simulink model "Outer_Loop_Autopilot"  (R2021b)
settings: Solver=FixedStepAuto  StartTime=0.0  StopTime=10.0  FixedStep=0.01  RelTol=1e-3
undefined symbols (not defined in the file): ap, uavParam
libraries: simulink x3, slpidlib x2, simulink_need_slupdate x1
settings Model: DataDictionary=stepFideltyResponseData.sldd  ModifiedByFormat=The MathWorks, Inc.  Creator=The MathWorks, Inc.  LastModifiedBy=The MathWorks, Inc.
settings DataIOCC: SaveOutput=off  SaveTime=off
settings OptimizationCC: UseDivisionForNetSlopeComputation=UseDivisionForReciprocalsOfIntegersOnly

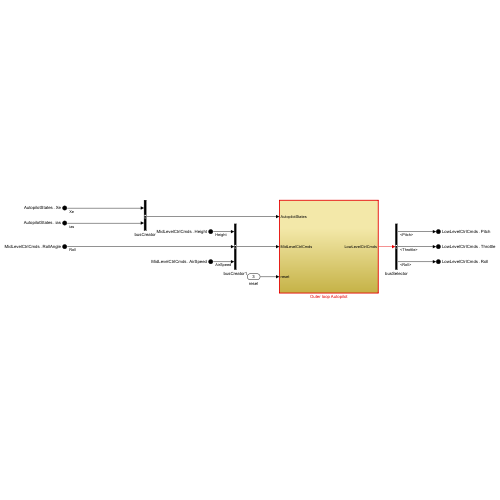
[thumbnail: Simulink's stored preview of the top-level diagram]
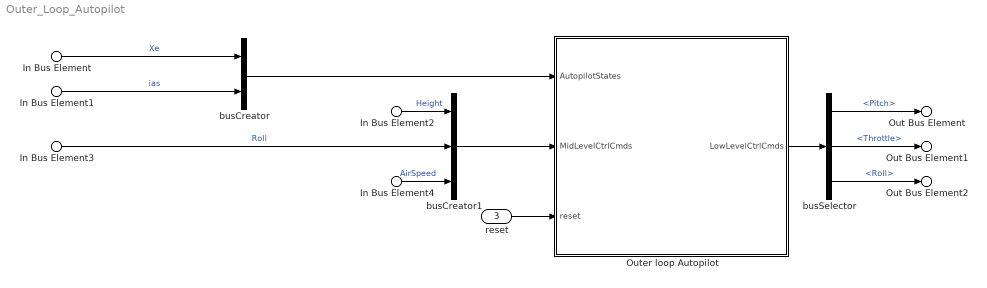
== system Outer_Loop_Autopilot ==
  In Bus Element : Inport  PortName=AutopilotStates  Element=Xe
  In Bus Element1 : Inport  PortName=AutopilotStates  Element=ias
  In Bus Element2 : Inport  Port=2  PortName=MidLevelCtrlCmds  Element=Height
  In Bus Element3 : Inport  Port=2  PortName=MidLevelCtrlCmds  Element=RollAngle
  In Bus Element4 : Inport  Port=2  PortName=MidLevelCtrlCmds  Element=AirSpeed
  reset : Inport  Port=3  OutDataTypeStr=double  PortDimensions=1  SampleTime=[0.01,0]
  Outer loop Autopilot : Subsystem  TreatAsAtomicUnit=on
  busCreator : BusCreator  Inputs=2
  busCreator1 : BusCreator  Inputs=3
  busSelector : BusSelector  OutputSignals=Pitch,Throttle,Roll
  Out Bus Element : Outport  PortName=LowLevelCtrlCmds  Element=Pitch
  Out Bus Element1 : Outport  PortName=LowLevelCtrlCmds  Element=Throttle
  Out Bus Element2 : Outport  PortName=LowLevelCtrlCmds  Element=Roll
  wires:
  busCreator1/1 -> Outer loop Autopilot/2(MidLevelCtrlCmds)
  Outer loop Autopilot/1(LowLevelCtrlCmds) -> busSelector/1
  In Bus Element/1 -> busCreator/1  "Xe"
  In Bus Element4/1 -> busCreator1/3  "AirSpeed"
  In Bus Element2/1 -> busCreator1/1  "Height"
  reset/1 -> Outer loop Autopilot/3(reset)
  In Bus Element3/1 -> busCreator1/2  "Roll"
  busCreator/1 -> Outer loop Autopilot/1(AutopilotStates)
  busSelector/1 -> Out Bus Element/1  "<Pitch>"
  busSelector/2 -> Out Bus Element1/1  "<Throttle>"
  busSelector/3 -> Out Bus Element2/1  "<Roll>"
  In Bus Element1/1 -> busCreator/2  "ias"

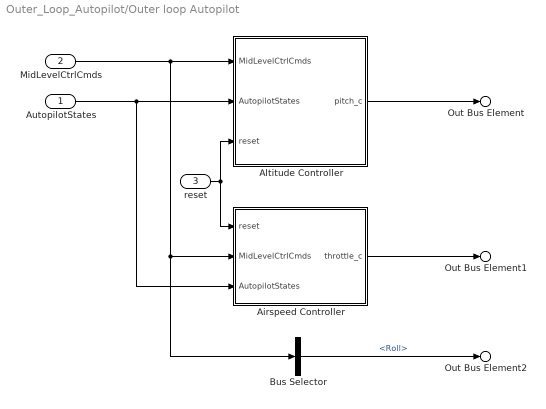
== system Outer_Loop_Autopilot/Outer loop Autopilot ==
  AutopilotStates : Inport
  MidLevelCtrlCmds : Inport  Port=2
  reset : Inport  Port=3
  Airspeed Controller : Subsystem  VariantControl=AirspeedCont~=1
  Altitude Controller : Subsystem  VariantControl=AltCont==0
  Bus Selector : BusSelector  OutputSignals=Roll
  Out Bus Element : Outport  PortName=LowLevelCtrlCmds  Element=Pitch
  Out Bus Element1 : Outport  PortName=LowLevelCtrlCmds  Element=Throttle
  Out Bus Element2 : Outport  PortName=LowLevelCtrlCmds  Element=Roll
  wires:
  Altitude Controller/1(pitch_c) -> Out Bus Element/1
  Airspeed Controller/1(throttle_c) -> Out Bus Element1/1
  Bus Selector/1 -> Out Bus Element2/1  "<Roll>"
  AutopilotStates/1 -> Altitude Controller/2(AutopilotStates), Airspeed Controller/3(AutopilotStates)
  MidLevelCtrlCmds/1 -> Airspeed Controller/2(MidLevelCtrlCmds), Bus Selector/1, Altitude Controller/1(MidLevelCtrlCmds)
  reset/1 -> Airspeed Controller/1(reset), Altitude Controller/3(reset)

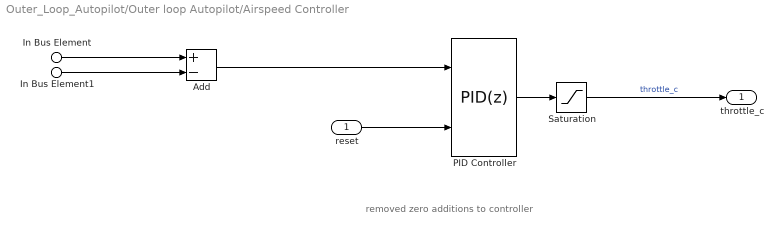
== system Outer_Loop_Autopilot/Outer loop Autopilot/Airspeed Controller ==
  note: removed zero additions to controller
  reset : Inport
  In Bus Element : Inport  Port=2  PortName=MidLevelCtrlCmds  Element=AirSpeed
  In Bus Element1 : Inport  Port=3  PortName=AutopilotStates  Element=ias
  Add : Sum  Inputs=+-
  PID Controller : slpidlib/PID Controller  Controller=PID  Form=Parallel  TimeDomain=Discrete-time  UseExternalTs=off  SampleTime=0.01  IntegratorMethod=Trapezoidal  FilterMethod=Forward Euler  ControllerParametersSource=internal  P=1.3  I=0.15  D=0  UseFilter=on  N=ap.control.derivativesConstant  TunerSelectOption=Transfer Function Based (PID Tuner App)  InitialConditionSource=internal  InitialConditionForIntegrator=0  InitialConditionForFilter=0  DifferentiatorICPrevScaledInput=0  ExternalReset=level  TrackingMode=off  Kt=1  LimitOutput=on  SatLimitsSource=internal  UpperSaturationLimit=ap.control.dtLimit  LowerSaturationLimit=0  LinearizeAsGain=on  AntiWindupMode=clamping  Kb=1  POutMin=[]  POutMax=[]  IOutMin=[]  IOutMax=[]  DOutMin=[]  DOutMax=[]  NOutMin=[]  NOutMax=[]  SumOutMin=[]  SumOutMax=[]  SaturationOutMin=[]  SaturationOutMax=[]  PParamMin=[]  PParamMax=[]  IParamMin=[]  IParamMax=[]  DParamMin=[]  DParamMax=[]  NParamMin=[]  NParamMax=[]  KbParamMin=[]  KbParamMax=[]  KtParamMin=[]  KtParamMax=[]  KbOutMin=[]  KbOutMax=[]  KtOutMin=[]  KtOutMax=[]  IntegratorOutMin=[]  IntegratorOutMax=[]  FilterOutMin=[]  FilterOutMax=[]  SumI1OutMin=[]  SumI1OutMax=[]  SumI2OutMin=[]  SumI2OutMax=[]  SumI3OutMin=[]  SumI3OutMax=[]  SumI4OutMin=[]  SumI4OutMax=[]  SumDOutMin=[]  SumDOutMax=[]  DifferentiatorOutMin=[]  DifferentiatorOutMax=[]  FilterDiffOutCoefMin=[]  FilterDiffOutCoefMax=[]  ReciprocalOutMin=[]  ReciprocalOutMax=[]  SumDenOutMin=[]  SumDenOutMax=[]  SumNumOutMin=[]  SumNumOutMax=[]  DivideOutMin=[]  DivideOutMax=[]  UdiffTsProdOutMin=[]  UdiffTsProdOutMax=[]  NTsProdOutMin=[]  NTsProdOutMax=[]  UintegralTsProdOutMin=[]  UintegralTsProdOutMax=[]  UngainTsProdOutMin=[]  UngainTsProdOutMax=[]  IntegratorContinuousStateAttributes=''  IntegratorStateMustResolveToSignalObject=off  IntegratorRTWStateStorageClass=Auto  FilterContinuousStateAttributes=''  FilterStateMustResolveToSignalObject=off  FilterRTWStateStorageClass=Auto  ParallelPVariant=InternalParameters  IdealPVariant=Disabled  IVariant=InternalParameters  DVariant=InternalParameters  IntegratorVariant=Discrete  SatVariant=Enabled  AWVariant=DiscClampingParallel  PCopyVariant=Disabled  TRVariant=Disabled  FdbkBlocksVariant=Feedback  IdealPFdbkVariant=Passthrough  SatFdbkVariant=Passthrough  DerivativeFilterVariant=ForwardEulerFilter  NVariant=InternalParameters  NCopyVariant=Disabled  FilterICVariant=InternalICsFilter  IntegratorICVariant=InternalICs  ExternalResetVariant=ExternalReset  TRSumVariant=Passthrough  SumFdbkVariant=Enabled  SumVariant=Sum_PID  TsampFilterVariant=InternalTs  TsampNgainVariant=Passthrough  TsampIntegralVariant=Passthrough  ExternalSaturationOutDataTypeStr=Inherit: Same as second input
  Saturation : Saturate  UpperLimit=ap.control.dtLimit  LowerLimit=0  OutDataTypeStr=double
  throttle_c : Outport
  wires:
  PID Controller/1 -> Saturation/1
  reset/1 -> PID Controller/2
  In Bus Element1/1 -> Add/2
  In Bus Element/1 -> Add/1
  Saturation/1 -> throttle_c/1  "throttle_c"
  Add/1 -> PID Controller/1

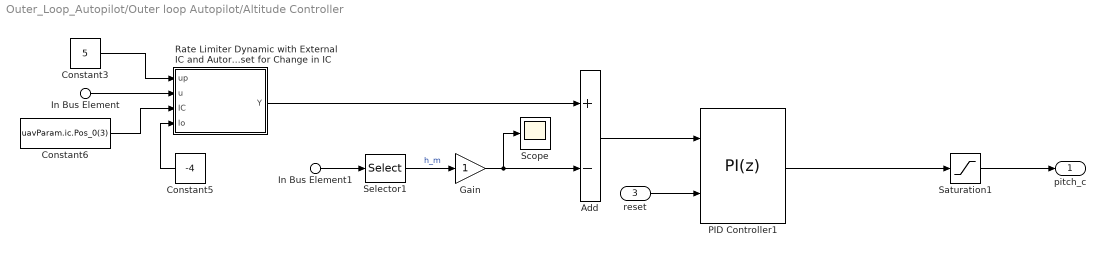
== system Outer_Loop_Autopilot/Outer loop Autopilot/Altitude Controller ==
  In Bus Element : Inport  PortName=MidLevelCtrlCmds  Element=Height
  In Bus Element1 : Inport  Port=2  PortName=AutopilotStates  Element=Xe
  reset : Inport  Port=3
  Add : Sum  Inputs=+-
  Constant3 : Constant  Value=5  OutDataTypeStr=Inherit: Inherit via back propagation
      settings: AttributesFormatString=%<Value>
  Constant5 : Constant  Value=-4  OutDataTypeStr=Inherit: Inherit via back propagation
      settings: AttributesFormatString=%<Value>
  Constant6 : Constant  Value=uavParam.ic.Pos_0(3)  OutDataTypeStr=double
      settings: AttributesFormatString=%<Value>
  Gain : Gain
  PID Controller1 : slpidlib/PID Controller  Controller=PI  Form=Parallel  TimeDomain=Discrete-time  UseExternalTs=off  SampleTime=ap.apSampleTime  IntegratorMethod=Trapezoidal  FilterMethod=Forward Euler  ControllerParametersSource=internal  P=0.05  I=0.001  D=0  UseFilter=on  N=5  TunerSelectOption=Transfer Function Based (PID Tuner App)  InitialConditionSource=internal  InitialConditionForIntegrator=0  InitialConditionForFilter=0  DifferentiatorICPrevScaledInput=0  ExternalReset=level  TrackingMode=off  Kt=1  LimitOutput=on  SatLimitsSource=internal  UpperSaturationLimit=ap.control.the_cLimit  LowerSaturationLimit=-ap.control.the_cLimit  LinearizeAsGain=on  AntiWindupMode=clamping  Kb=1  POutMin=[]  POutMax=[]  IOutMin=[]  IOutMax=[]  DOutMin=[]  DOutMax=[]  NOutMin=[]  NOutMax=[]  SumOutMin=[]  SumOutMax=[]  SaturationOutMin=[]  SaturationOutMax=[]  PParamMin=[]  PParamMax=[]  IParamMin=[]  IParamMax=[]  DParamMin=[]  DParamMax=[]  NParamMin=[]  NParamMax=[]  KbParamMin=[]  KbParamMax=[]  KtParamMin=[]  KtParamMax=[]  KbOutMin=[]  KbOutMax=[]  KtOutMin=[]  KtOutMax=[]  IntegratorOutMin=[]  IntegratorOutMax=[]  FilterOutMin=[]  FilterOutMax=[]  SumI1OutMin=[]  SumI1OutMax=[]  SumI2OutMin=[]  SumI2OutMax=[]  SumI3OutMin=[]  SumI3OutMax=[]  SumI4OutMin=[]  SumI4OutMax=[]  SumDOutMin=[]  SumDOutMax=[]  DifferentiatorOutMin=[]  DifferentiatorOutMax=[]  FilterDiffOutCoefMin=[]  FilterDiffOutCoefMax=[]  ReciprocalOutMin=[]  ReciprocalOutMax=[]  SumDenOutMin=[]  SumDenOutMax=[]  SumNumOutMin=[]  SumNumOutMax=[]  DivideOutMin=[]  DivideOutMax=[]  UdiffTsProdOutMin=[]  UdiffTsProdOutMax=[]  NTsProdOutMin=[]  NTsProdOutMax=[]  UintegralTsProdOutMin=[]  UintegralTsProdOutMax=[]  UngainTsProdOutMin=[]  UngainTsProdOutMax=[]  IntegratorContinuousStateAttributes=''  IntegratorStateMustResolveToSignalObject=off  IntegratorRTWStateStorageClass=Auto  FilterContinuousStateAttributes=''  FilterStateMustResolveToSignalObject=off  FilterRTWStateStorageClass=Auto  ParallelPVariant=InternalParameters  IdealPVariant=Disabled  IVariant=InternalParameters  DVariant=Disabled  IntegratorVariant=Discrete  SatVariant=Enabled  AWVariant=DiscClampingParallel  PCopyVariant=Disabled  TRVariant=Disabled  FdbkBlocksVariant=Feedback  IdealPFdbkVariant=Passthrough  SatFdbkVariant=Passthrough  DerivativeFilterVariant=Disabled  NVariant=Disabled  NCopyVariant=Disabled_SignalSpec  FilterICVariant=Disabled  IntegratorICVariant=InternalICs  ExternalResetVariant=ExternalReset  TRSumVariant=Passthrough  SumFdbkVariant=Enabled  SumVariant=Sum_PI  TsampFilterVariant=InternalTs  TsampNgainVariant=Passthrough  TsampIntegralVariant=Passthrough  ExternalSaturationOutDataTypeStr=Inherit: Same as second input
  Rate Limiter Dynamic with External IC and Autoreset for Change in IC : Subsystem
      mask Display:
      | plot([0.15 0.95],[.5 .5],[.5 .5],[0.05 0.95],0.05+0.9*[.2 .8],0.05+0.9*[0 1]);
      | port_label('output',1,'Y');
      | port_label('input',1,'up');
      | port_label('input',2,'u');
      | port_label('input',3,'IC');
      | port_label('input',4,'Lo');
  Saturation1 : Saturate  UpperLimit=ap.control.the_cLimit  LowerLimit=-ap.control.the_cLimit  OutDataTypeStr=double
  Scope : Scope
  Selector1 : Selector  InputPortWidth=3  IndexOptions=Index vector (dialog)  Indices=[3]  OutputSizes=1
  pitch_c : Outport
  wires:
  Selector1/1 -> Gain/1  "h_m"
  Rate Limiter Dynamic with External IC and Autoreset for Change in IC/1(Y) -> Add/1
  reset/1 -> PID Controller1/2
  PID Controller1/1 -> Saturation1/1
  Add/1 -> PID Controller1/1
  Constant6/1 -> Rate Limiter Dynamic with External IC and Autoreset for Change in IC/3(IC)
  In Bus Element/1 -> Rate Limiter Dynamic with External IC and Autoreset for Change in IC/2(u)
  Constant3/1 -> Rate Limiter Dynamic with External IC and Autoreset for Change in IC/1(up)
  Constant5/1 -> Rate Limiter Dynamic with External IC and Autoreset for Change in IC/4(lo)
  In Bus Element1/1 -> Selector1/1
  Gain/1 -> Add/2, Scope/1
  Saturation1/1 -> pitch_c/1

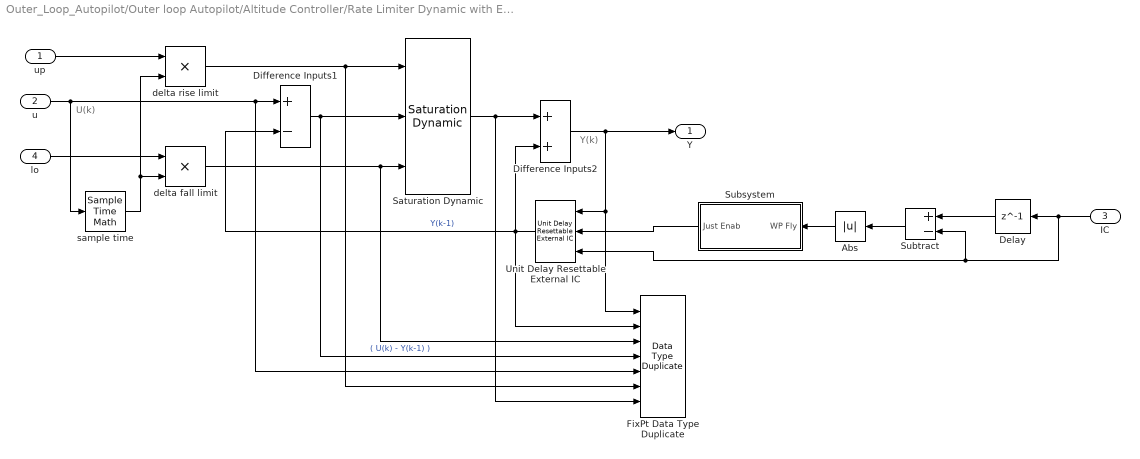
== system Outer_Loop_Autopilot/Outer loop Autopilot/Altitude Controller/Rate Limiter Dynamic with External IC and Autoreset for Change in IC ==
  note: U(k)
  note: Y(k)
  up : Inport
  u : Inport  Port=2
  IC : Inport  Port=3
  lo : Inport  Port=4
  Abs : Abs
  Delay : Delay  DelayLength=1
  Difference Inputs1 : Sum  Description=Add in CPU  DisableCoverage=on  Inputs=+-  OutDataTypeStr=Inherit: Inherit via back propagation
  Difference Inputs2 : Sum  Description=Add in CPU  OutDataTypeStr=Inherit: Inherit via back propagation
  FixPt Data Type Duplicate : DataTypeDuplicate  DisableCoverage=on  NumInputPorts=7
  Saturation Dynamic : simulink/Discontinuities/Saturation Dynamic  OutMin=[]  OutMax=[]  OutDataTypeStr=Inherit: Same as second input  OutDataType=fixdt(1, 16)  OutScaling=2^-10  DoSatur=off
  Subsystem : Subsystem
  Subtract : Sum  Inputs=+-
  Unit Delay Resettable External IC : simulink_need_slupdate/Unit Delay Resettable External IC  tsamp=-1
      settings: SourceProductBaseCode=SL
  delta fall limit : Product  DisableCoverage=on  Inputs=**  OutDataTypeStr=Inherit: Inherit via back propagation  SaturateOnIntegerOverflow=on
  delta rise limit : Product  DisableCoverage=on  Inputs=**  OutDataTypeStr=Inherit: Inherit via back propagation  SaturateOnIntegerOverflow=on
  sample time : SampleTimeMath  DisableCoverage=on  TsampMathOp=Ts Only  weightValue=1
  Y : Outport  VectorParamsAs1DForOutWhenUnconnected=off
  wires:
  Difference Inputs1/1 -> Saturation Dynamic/2, FixPt Data Type Duplicate/4  "( U(k) - Y(k-1) )"
  u/1 -> sample time/1, FixPt Data Type Duplicate/5, Difference Inputs1/1
  delta fall limit/1 -> Saturation Dynamic/3, FixPt Data Type Duplicate/3
  Saturation Dynamic/1 -> FixPt Data Type Duplicate/7, Difference Inputs2/1
  Unit Delay Resettable External IC/1 -> Difference Inputs2/2, FixPt Data Type Duplicate/2, Difference Inputs1/2  "Y(k-1)"
  Difference Inputs2/1 -> Y/1, Unit Delay Resettable External IC/1, FixPt Data Type Duplicate/1
  up/1 -> delta rise limit/1
  delta rise limit/1 -> Saturation Dynamic/1, FixPt Data Type Duplicate/6
  lo/1 -> delta fall limit/1
  sample time/1 -> delta rise limit/2, delta fall limit/2
  Delay/1 -> Subtract/1
  IC/1 -> Unit Delay Resettable External IC/3, Subtract/2, Delay/1
  Subtract/1 -> Abs/1
  Subsystem/1(Just Enab) -> Unit Delay Resettable External IC/2
  Abs/1 -> Subsystem/1(WP Fly)

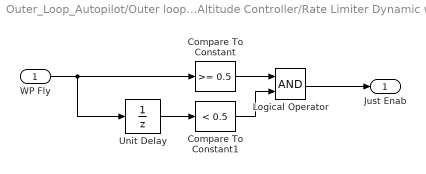
== system Outer_Loop_Autopilot/Outer loop Autopilot/Altitude Controller/Rate Limiter Dynamic with External IC and Autoreset for Change in IC/Subsystem ==
  WP Fly : Inport
  Compare To Constant : simulink/Logic and Bit Operations/Compare To Constant  relop=>=  const=0.5  OutDataTypeStr=boolean
  Compare To Constant1 : simulink/Logic and Bit Operations/Compare To Constant  relop=<  const=0.5  OutDataTypeStr=boolean
  Logical Operator : Logic  AllPortsSameDT=off  OutDataTypeStr=boolean
  Unit Delay : UnitDelay  SampleTime=-1  HasFrameUpgradeWarning=on
  Just Enab : Outport  VectorParamsAs1DForOutWhenUnconnected=off
  wires:
  Logical Operator/1 -> Just Enab/1
  Unit Delay/1 -> Compare To Constant1/1
  Compare To Constant1/1 -> Logical Operator/2
  Compare To Constant/1 -> Logical Operator/1
  WP Fly/1 -> Compare To Constant/1, Unit Delay/1
